simulink model "VisualizationData_Faulty"  (R2020a)
settings: Solver=VariableStepAuto  StartTime=0.0  StopTime=60  RelTol=1e-3
settings Model: Creator=kashy  LastModifiedBy=kashy

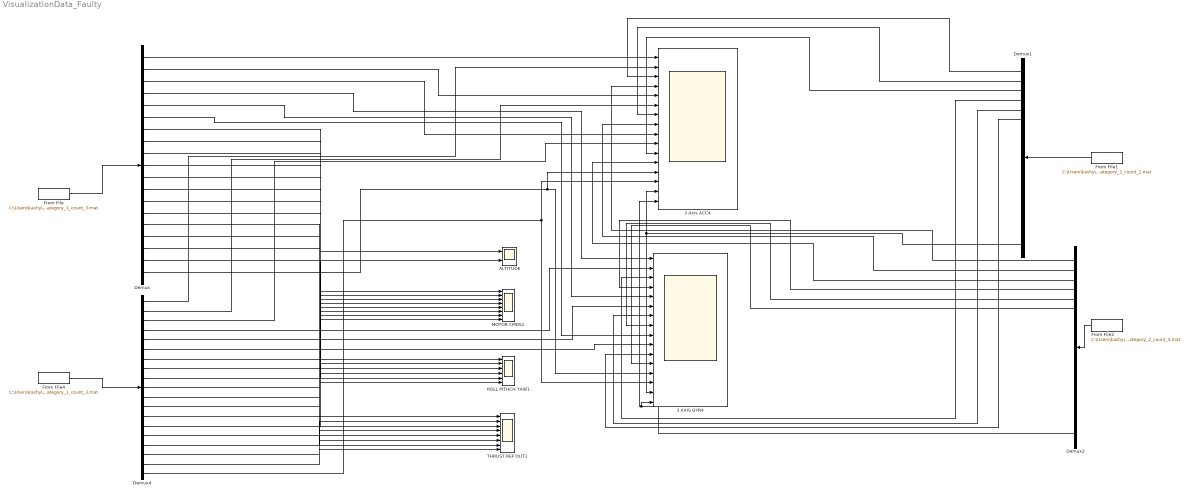
== system VisualizationData_Faulty ==
  3 AXIS GYR4 : Scope  NumInputPorts=16
  3 Axis ACC4 : Scope  NumInputPorts=16
  ALTITUDE : Scope  NumInputPorts=2
  Demux{,1..2,4} (4 alike) : Demux  Outputs=19
  From File : FromFile  FileName=C:\Users\kashy\Documents\MATLAB\Master_Thesis\model\parrotMinidroneWaypointFollower\FaultyDataGyr_MATFILES\1_Offset\Faulty_Simulation_wp_2_Fault_Category_1_count_3.mat  SampleTime=0.1
  From File1 : FromFile  FileName=C:\Users\kashy\Documents\MATLAB\Master_Thesis\model\parrotMinidroneWaypointFollower\FaultyDataAcc_MATFILES\2_Stuck_at\Faulty_Simulation_wp_9_Fault_Category_2_count_1.mat  SampleTime=0.01
  From File2 : FromFile  FileName=C:\Users\kashy\Documents\MATLAB\Master_Thesis\model\parrotMinidroneWaypointFollower\FaultyDataAcc_MATFILES\2_Stuck_at\Faulty_Simulation_wp_14_Fault_Category_2_count_3.mat  SampleTime=0.01
  From File4 : FromFile  FileName=C:\Users\kashy\Documents\MATLAB\Master_Thesis\model\parrotMinidroneWaypointFollower\FaultyDataGyr_MATFILES\1_Offset\Faulty_Simulation_wp_20_Fault_Category_1_count_3.mat  SampleTime=0.1
  MOTOR CMDS1 : Scope  NumInputPorts=8
  ROLL PITHCH YAW1 : Scope  NumInputPorts=6
  THRUST REF OUT1 : Scope  NumInputPorts=8
  wires:
  From File/1 -> Demux/1
  Demux/7 -> ALTITUDE/1
  From File4/1 -> Demux4/1
  Demux4/7 -> ALTITUDE/2
  Demux/8 -> MOTOR CMDS1/1
  Demux4/8 -> MOTOR CMDS1/2
  Demux/9 -> MOTOR CMDS1/3
  Demux4/9 -> MOTOR CMDS1/4
  Demux/10 -> MOTOR CMDS1/5
  Demux4/10 -> MOTOR CMDS1/6
  Demux/11 -> MOTOR CMDS1/7
  Demux4/11 -> MOTOR CMDS1/8
  Demux/12 -> ROLL PITHCH YAW1/1
  Demux4/12 -> ROLL PITHCH YAW1/2
  Demux/13 -> ROLL PITHCH YAW1/3
  Demux4/13 -> ROLL PITHCH YAW1/4
  Demux/14 -> ROLL PITHCH YAW1/5
  Demux4/14 -> ROLL PITHCH YAW1/6
  Demux/15 -> THRUST REF OUT1/1
  Demux4/15 -> THRUST REF OUT1/2
  Demux/16 -> THRUST REF OUT1/3
  Demux4/16 -> THRUST REF OUT1/4
  Demux/17 -> THRUST REF OUT1/5
  Demux4/17 -> THRUST REF OUT1/6
  Demux/18 -> THRUST REF OUT1/7
  Demux4/18 -> THRUST REF OUT1/8
  From File1/1 -> Demux1/1
  From File2/1 -> Demux2/1
  Demux/1 -> 3 Axis ACC4/1
  Demux4/1 -> 3 Axis ACC4/2
  Demux1/1 -> 3 Axis ACC4/3
  Demux2/1 -> 3 Axis ACC4/4
  Demux/2 -> 3 Axis ACC4/5
  Demux4/2 -> 3 Axis ACC4/6
  Demux1/2 -> 3 Axis ACC4/7
  Demux2/2 -> 3 Axis ACC4/8
  Demux/3 -> 3 Axis ACC4/9
  Demux4/3 -> 3 Axis ACC4/10
  Demux1/3 -> 3 Axis ACC4/11
  Demux2/3 -> 3 Axis ACC4/12
  Demux/19 -> 3 AXIS GYR4/13, 3 Axis ACC4/13
  Demux4/19 -> 3 AXIS GYR4/14, 3 Axis ACC4/14
  Demux1/19 -> 3 Axis ACC4/15, 3 AXIS GYR4/15
  Demux2/19 -> 3 AXIS GYR4/16, 3 Axis ACC4/16
  Demux/4 -> 3 AXIS GYR4/1
  Demux4/4 -> 3 AXIS GYR4/2
  Demux1/4 -> 3 AXIS GYR4/3
  Demux2/4 -> 3 AXIS GYR4/4
  Demux/5 -> 3 AXIS GYR4/5
  Demux4/5 -> 3 AXIS GYR4/6
  Demux1/5 -> 3 AXIS GYR4/7
  Demux2/5 -> 3 AXIS GYR4/8
  Demux/6 -> 3 AXIS GYR4/9
  Demux4/6 -> 3 AXIS GYR4/10
  Demux1/6 -> 3 AXIS GYR4/11
  Demux2/6 -> 3 AXIS GYR4/12
